simulink model "on_line_dyskretny_18"  (R2018a)
settings: Solver=VariableStepAuto  StartTime=0.0  StopTime=20  RelTol=1e-3
libraries: ctrlSharedLib x1
settings Model: Creator=Dominik  LastModifiedBy=a.kuligowski

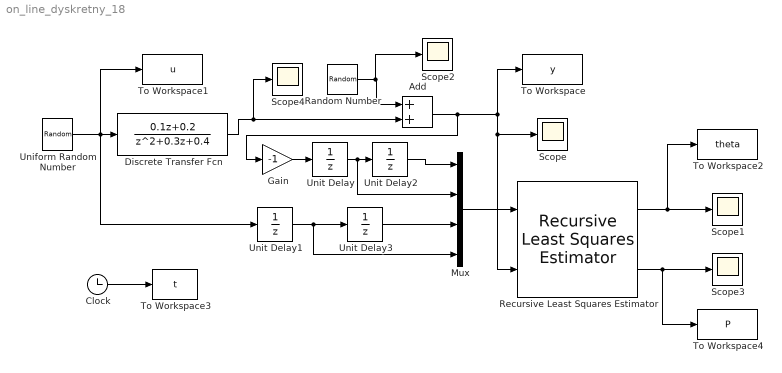
== system on_line_dyskretny_18 ==
  Add : Sum
  Clock : Clock
  Discrete Transfer Fcn : DiscreteTransferFcn  Numerator=[0.1 0.2]  Denominator=[1 0.3 0.4]
  Gain : Gain  Gain=-1
  Mux : Mux
  Random Number : RandomNumber  Variance=0.0006  Seed=3423  SampleTime=0.1
  Recursive Least Squares Estimator : ctrlSharedLib/Recursive Least Squares Estimator  InitialEstimateSource=None  InitialParameterData=4  P0=10  InitialRegressors=0  InitialOutputs=0  History=Infinite  WindowLength=200  EstimationMethod=Forgetting Factor  AdaptationParameter=1  HasTimeVaryingAdaptationParameter=off  NormalizationBias=eps  OutputError=off  OutputP=on  AddEnablePort=off  InputProcessing=Sample-based  Ts=-1
      settings: SourceProductName=Control System Toolbox  SourceProductBaseCode=CT
  Scope{,1..4} (5 alike) : Scope
  To Workspace : ToWorkspace  VariableName=y  SampleTime=-1
  To Workspace1 : ToWorkspace  VariableName=u  SampleTime=-1
  To Workspace2 : ToWorkspace  VariableName=theta  SampleTime=-1
  To Workspace3 : ToWorkspace  VariableName=t  SampleTime=-1
  To Workspace4 : ToWorkspace  VariableName=P  SampleTime=-1
  Uniform Random Number : UniformRandomNumber  SampleTime=0.1
  Unit Delay{,1..3} (4 alike) : UnitDelay  SampleTime=-1  HasFrameUpgradeWarning=on
  wires:
  Discrete Transfer Fcn/1 -> Scope4/1, Add/2
  Gain/1 -> Unit Delay/1
  Unit Delay/1 -> Mux/2, Unit Delay2/1
  Unit Delay1/1 -> Mux/4, Unit Delay3/1
  Uniform Random Number/1 -> Discrete Transfer Fcn/1, To Workspace1/1, Unit Delay1/1
  Mux/1 -> Recursive Least Squares Estimator/1
  Recursive Least Squares Estimator/1 -> To Workspace2/1, Scope1/1
  Clock/1 -> To Workspace3/1
  Recursive Least Squares Estimator/2 -> Scope3/1, To Workspace4/1
  Unit Delay2/1 -> Mux/1
  Unit Delay3/1 -> Mux/3
  Random Number/1 -> Scope2/1, Add/1
  Add/1 -> Gain/1, To Workspace/1, Recursive Least Squares Estimator/2, Scope/1
